simulink model "EvPowertrainController4EM"  (R2024b)
settings: configuration reference "VehicleFixed10ms" (kept outside this file)
model workspace (MAT data in the model file):
  CtrlVcuAccelPdlBpts = [0 0.8 1]
  CtrlVcuBattPnlty = 10000000
  CtrlVcuBattSOCBpts = [0 20 60 80 100]
  CtrlVcuCnstrntPnltyFctr = 10000000
  CtrlVcuEMPnlty = 100
  CtrlVcuEMTrqSplitGrid = 200
  CtrlVcuFallRate = -500
  CtrlVcuMaxAccelG = 1
  CtrlVcuMaxDecelG = -1.5
  CtrlVcuPwrDeltaPnlty = 50
  CtrlVcuPwrRatePnlty = [25 25 100]
  CtrlVcuRiseRate = 500
  CtrlVcuRoadMuEst = 0.8
  CtrlVcuSftyFctr = 0.9
  CtrlVcuTracPwrErrPnlty = 25
  CtrlVcuTrqVecBrkThresh = 0.01
  CtrlVcuTrqVecIGain = 0
  CtrlVcuTrqVecMinTrq = 25
  CtrlVcuTrqVecPGain = -2000
  CtrlVcuTrqVecSteerThresh = 0.349065850399
  CtrlVcuTrqVecVelThresh = 2.5
  N_P0 = 3
undefined symbols (not defined in the file): CtrlBcuTrlrBrkGain, CtrlVcuEvChrgLmtBpt, CtrlVcuEvRegenBrkCutOff, CtrlVcuEvRegenBrkSpdBpt, CtrlVcuEvSocBpt, eff, EnvGrvty, PlntBrkActrBoreFrnt, PlntBrkFrntBias, PlntBrkKinFricCffFrnt, PlntBrkNumPadsFrnt, PlntBrkPadMeanRadiusFrnt, PlntBrkPrsFctr, PlntBrkRearBias, PlntDiffrntl2Eff, PlntDiffrntl2Ratio, PlntDiffrntlEff, PlntDiffrntlRatio, PlntEM1EffTbl, PlntEM1Spd, PlntEM1SpdEff, PlntEM1Trq, PlntEM1TrqEff, PlntEM2EffTbl, PlntEM2Spd, PlntEM2SpdEff, PlntEM2Trq, PlntEM2TrqEff, PlntEM3EffTbl, PlntEM3Spd, PlntEM3SpdEff, PlntEM3Trq, PlntEM3TrqEff, PlntEMWhlGearEffFL, PlntEMWhlGearEffRL, PlntEMWhlGearRatioFL, PlntEMWhlGearRatioRL, PlntTransEffSpdBpt, PlntTransEffTbl, PlntTransEffTempBpt, PlntTransEffTrqBpt, PlntTransGearNumVect, PlntTransGearRatioVect, PlntVehCGHgtAxl, PlntVehDstCGFrntAxl, PlntVehDstCGRearAxl, PlntVehMass, PlntWhlLdRadiusFrnt, PlntWhlLdRadiusRear
libraries: simulink x25, autolibutils x2, slpidlib x2
(part 7 of 7)

== matlab function EvPowertrainController4EM/Torque Vectoring/Nonlinear_MPC/Nonlinear_MPCFcn ==
  data: Acc input; delta_Frnt input; TV_enableflag input; xk input; PrevEMTrqCmdFinals input; EMTrqCmds input; Vx input; EMTrqMaxFrnt input; EMTrqMaxRear input; xi_in input; EMTrqCmdFinal output; xhat_kp1 output; fval output; exitflag output; allCosts output; compTime output; stepSize output; iterations output; funcCount output; betaMax output; r_ref output; xi_out output
function [EMTrqCmdFinal, xhat_kp1, fval, exitflag, allCosts, compTime, stepSize, iterations, funcCount, betaMax, r_ref, xi_out] ...
    = Nominal_MPC(Acc, delta_Frnt, TV_enableflag, xk, PrevEMTrqCmdFinals, EMTrqCmds, Vx, EMTrqMaxFrnt, EMTrqMaxRear, xi_in)

%% MPC Tuning Parameters
Np = 10;    % prediction horizon [interval]
Nc = 3;     % control horizon [interval] 

% % -----------------------------------------------------------------

Q_y  = 150;     % Weight of yaw rate tracking
Q_du = eye(4);  % Weight of input increment (slew rate)

% % -----------------------------------------------------------------

% % % Allowed Maximum NMPC computation Iterations
Iter_max = 30;

%% Defining fixed parameter structure
nx = 2; % number of states
nu = 2; % number of controls

% % System parameters
m  = 1623;          % [kg]           % vehicle mass
Iz = 2066;          % [kg m^2]       % yaw moment of inertia
lf = 1.09;          % [m]            % distance from c.o.g. to front axle
lr = 1.7;           % [m]            % distance from c.o.g. to rear axle
lw = 1.575;         % [m]            % track width
rw = 0.309;         % [m]            % wheel radius
h  = 0.609;         % [m]            % distance from c.o.g. to ground
g  = 9.81;          % [m/s^2]        % gravitational acceleration

mu_x = 0.8*0.9;     % assumed tire-road friction coefficient

% % Tires' magic formula coefficients
D = 1.0;    % []            % peak factor scale
C = 1.1;    % []            % shape factor
E = 1.2;    % []            % curvature factor

EMWhlGearRatio = 0.98*4.1; % (wheel torque = efficiency * 4.1 * motor torque)

EMTrqIncMax = 500*0.01.*ones(4,1); % sampling time = 0.01 [s];

EMFrntTrq = EMTrqCmds(1) + EMTrqCmds(2); % front axle (motor) torque
EMRearTrq = EMTrqCmds(3) + EMTrqCmds(4); % rear  axle (motor) torque

%% System bounds
% % Bounds on input and state
u_max = [2*EMTrqMaxFrnt; 2*EMTrqMaxRear];
x_max = [Inf; Inf]; % No bounds

% % % Upper Bound on Decision Variables
xi_max = [kron(ones(Nc,1), u_max);    % control
          kron(ones(Np,1), x_max)];  % states

% % Lower Bound on Decision Variables
xi_min = [kron(ones(Nc,1), -u_max);    % control
          kron(ones(Np,1), -x_max)];  % states

% % Maximum side slip angle
Car = 2.4E4; % (estimated) rear cornering stiffness
betaMax = abs(mu_x*g*(lr/Vx^2 + m*lf/(Car*(lf+lr))));

%% Yaw rate reference
% Neutral steer
r_ref = Vx*delta_Frnt/(lf+lr);

% Maximum yaw rate reference
r_ref_max = abs(0.85* mu_x*g/Vx); 

% Saturated reference
if abs(r_ref) > r_ref_max
    r_ref = r_ref_max*sign(delta_Frnt);
end

%% Provide an initial guess by shifting the previous solution 1 step (Warm Start)
% Calculate indices for clarity
% Controls
control_end = nu*Nc;
% States
state_end   = control_end + nx*Np;

% Construct the warm start vector by shifting previous solution
xi_0 = [xi_in(nu+1 : control_end);              % shifted controls (skip first control)
        xi_in(control_end-nu+1 : control_end);  % repeat last control
        xi_in(control_end+nx+1 : state_end);    % shifted states (skip first state)
        xi_in(state_end-nx+1 : state_end)];      % repeat last state

%% Fixed parameter structure
params = struct('m',m,'Iz',Iz,'lf',lf,'lr',lr,'lw',lw,'rw',rw,'h',h,'g',g, ...
    'D', D, 'C', C, 'E', E, ...
    'Np',Np,'Nc',Nc, ...
    'Q_y',Q_y,'Q_du',Q_du, ...
    'mu_x',mu_x, 'EMTrqIncMax', EMTrqIncMax, 'EMWhlGearRatio',EMWhlGearRatio, ...
    'control_end', control_end, 'state_end', state_end);

%% MPC Call

% % Solver settings
nmpc_options = optimoptions('fmincon', 'Algorithm', 'sqp', 'MaxIterations',Iter_max, 'ScaleProblem',true);

% % % If Torque Vectoring is enable, use MPC
if TV_enableflag > 0.5

    timeStart = tic;
    [xi_out, fval, exitflag, output] = fmincon(@(xi_seq) sum(MPC_getCosts(xi_seq, xk, PrevEMTrqCmdFinals, ...
                                                EMFrntTrq, EMRearTrq, r_ref, params)),...
             xi_0, ...
             [], ...          % 
             [], ...          % 
             [], ...          % 
             [], ...          % 
             xi_min, ...
             xi_max, ...
             @(xi_seq) MPC_getConstraints(xi_seq, xk, PrevEMTrqCmdFinals, Vx, delta_Frnt, ...
                                EMTrqMaxFrnt, EMTrqMaxRear, Acc, EMFrntTrq, EMRearTrq, params), ...
             nmpc_options);

    compTime = toc(timeStart); % 0        
    % NOTE: Using tic-toc to measure computation time ONLY IF NECESSARY
    % MATLAB advises not to use tic-toc with code generation.
    % tic-toc code gen is different from the normal MATLAB code gen. 
    % They later cause problems for other control variants (PID subsystem and No Torque Vectoring subsystem)  
    
    % % Extract optimal controls
    EMTrqCmdFinal = getEMTrqs(EMFrntTrq, EMRearTrq, xi_out(1:nu));

    % % Obtain optimal (predicted) next state
    xhat_kp1 = MPC_getNextState(xk, xi_out(1:nu), EMFrntTrq, Vx, delta_Frnt, Acc, params);

    % % Acquire computed costs to examine the influence of different costs 
    allCosts = MPC_getCosts(xi_out, xk, PrevEMTrqCmdFinals, EMFrntTrq, EMRearTrq, r_ref, params);
    
    % % Last Step length by sqp
    stepSize = output.lssteplength;
    
    % % Iterations taken by fmincon
    iterations = output.iterations;

    % % Number of function evaluations
    funcCount = output.funcCount;

else    % if Torque Vectoring is not enable, use default torque commands
    EMTrqCmdFinal = EMTrqCmds;

    xi_out      = [kron(ones(Nc,1), [0;0]); % control
                   kron(ones(Np,1), xk)];      % states

    xhat_kp1    = xk;
    allCosts    = [0;0];
    exitflag    = 0;
    fval        = 0;
    compTime    = 0;
    stepSize    = 0;
    iterations  = 0;
    funcCount   = 0;
end

% % % --------------------- end of main program ----------------------


% % % ----------------------- begin of costs -----------------------

%% Cost Function
function J_vec = MPC_getCosts(xi_seq, x0, PrevEMTrqCmdFinals, EMFrntTrq, EMRearTrq, r_ref, params)
    % % Dimensions
    nx = 2;
    nu = 2;
    Nc = params.Nc;
    Np = params.Np;

    % % Initialization
    J_y         = 0;        % cost of yaw rate tracking
    J_du        = 0;        % cost of torque increment (slew rate)

    % % Extract and reshape controls from column vector (nu*Nc, 1) to matrix (nu, Nc)
    u_seq = reshape(xi_seq(1 : params.control_end), nu, Nc);

    % % Extract and reshape state sequence
    x_seq = reshape(xi_seq(params.control_end+1 : params.state_end), nx, Np);
    
    % Yaw rate tracking
    % J_y = J_y + params.Q_y*(x0(2) - r_ref)^2;
    for k = 1 : Np-1
        % Yaw rate tracking
        J_y = J_y + params.Q_y*(x_seq(2,k) - r_ref)^2;
    end
    
    % % Torque increment
    TrqInc = getEMTrqs(EMFrntTrq, EMRearTrq, u_seq(:,1)) - PrevEMTrqCmdFinals;
    J_du = J_du + TrqInc.' * params.Q_du  * TrqInc;
    %
    for k = 2 : Nc
        TrqInc = getEMTrqs(EMFrntTrq, EMRearTrq, u_seq(:,k)) ...
                    - getEMTrqs(EMFrntTrq, EMRearTrq, u_seq(:,k-1));
        J_du = J_du + TrqInc.' * params.Q_du  * TrqInc;
    end

    % % Cost vector
    J_vec = [J_y; J_du];

% end

% % % --------------------- end of costs ----------------------

% % % --------------------- begin of constraints -----------------------

%% Constraint function
function [c_ineq, c_eq] = MPC_getConstraints(xi_seq, x0, PrevEMTrqCmdFinals, ...
    Vx, delta_Frnt, EMTrqMaxFrnt, EMTrqMaxRear, Acc, EMFrntTrq, EMRearTrq, params)
    % % Dimensions
    nx = 2;
    nu = 2;
    Nc = params.Nc;
    Np = params.Np;

    % % Extract and reshape controls from column vector (nu*Nc, 1) to matrix (nu, Nc)
    u_seq = reshape(xi_seq(1 : params.control_end), nu, Nc);

    % % Extract and reshape state sequence
    x_seq = reshape(xi_seq(params.control_end+1 : params.state_end), nx, Np);
    
    % % Torque increment sequence
    EMTrqs_seq = zeros(4, Nc);
    for k = 1 : Nc
        EMTrqs_seq(:,k) = getEMTrqs(EMFrntTrq, EMRearTrq, u_seq(:,k));
    end
    EMTrqInc_seq = [EMTrqs_seq(:,1)-PrevEMTrqCmdFinals, diff(EMTrqs_seq,1,2)];

    % % -----------------------------------------------------------------
    % % % % State Continuity (SC) constraints
    c_eq_SC = nan(nx*Np,1);
    
    % State propagation
    xkp1 = MPC_getNextState(x0, u_seq(:,1), EMFrntTrq, Vx, delta_Frnt, Acc, params);
    % Continuity constraint
    c_eq_SC(1 : nx) = x_seq(:,1) - xkp1;

    for k = 2 : 1 : Nc
        % State propagation
        xkp1 = MPC_getNextState(x_seq(:,k-1), u_seq(:,k), EMFrntTrq, Vx, delta_Frnt, Acc, params);
        % Continuity constraint
        c_eq_SC(nx*(k-1)+1 : nx*(k-1)+nx) = x_seq(:,k) - xkp1;
    end

    for k = Nc+1 : 1 : Np
        % State propagation
        xkp1 = MPC_getNextState(x_seq(:,k-1), u_seq(:,Nc), EMFrntTrq, Vx, delta_Frnt, Acc, params);
        % Continuity constraint
        c_eq_SC(nx*(k-1)+1 : nx*(k-1)+nx) = x_seq(:,k) - xkp1;
    end

    % % -----------------------------------------------------------------
    % % Pure-control inequality constraint  
    c_ineq_EMTrqIncMax = nan(2*4*Nc,1); % % % Torque increment bound constraints
    c_ineq_EMTrqsMax = nan(2*4*Nc,1);  % % % Maximum allowed torque constraints
    c_ineq_vecTrq = nan(2*Nc, 1); % % % Torque vectoring encouraging constraints

    EMTrqsMax = [EMTrqMaxFrnt; EMTrqMaxFrnt; EMTrqMaxRear; EMTrqMaxRear];

    for k = 1 : Nc
        % % Maximum allowed torque increment Constraints
        c_ineq_EMTrqIncMax(2*4*(k-1)+1 : 2*4*(k-1)+2*4) = [ EMTrqInc_seq(:,k) - params.EMTrqIncMax;
                                                           -EMTrqInc_seq(:,k) - params.EMTrqIncMax ];
        % % Maximum allowed torque Constraints
        c_ineq_EMTrqsMax(2*4*(k-1)+1:2*4*(k-1)+2*4) = [ EMTrqs_seq(:,k) - EMTrqsMax;
                                                       -EMTrqs_seq(:,k) - EMTrqsMax];
        % % Vectoring torque encouragement
        c_ineq_vecTrq(2*(k-1)+1 : 2*(k-1)+2) = [-u_seq(1,k)*delta_Frnt;
                                                -u_seq(2,k)*delta_Frnt];

    end
    
    % % -----------------------------------------------------------------
    % % Inequality constraints
    c_ineq = [c_ineq_EMTrqIncMax;
              c_ineq_EMTrqsMax;
              c_ineq_vecTrq];

    % % Equality constraint
    c_eq = c_eq_SC;

% end

% % % --------------------- end of constraints ----------------------

% % % --------------------- begin of dynamics ----------------------

function xkp1 = MPC_getNextState(xk, uk, EMFrntTrq, Vx, delta_Frnt, Acc, params)
Ts = 0.01;

% % % 4th order
% k1 = MPC_getVehicleDynamics(xk, uk, EMFrntTrq, Vx, delta_Frnt, Acc, params);
% k2 = MPC_getVehicleDynamics(xk + Ts*k1/2, uk, EMFrntTrq, Vx, delta_Frnt, Acc, params);
% k3 = MPC_getVehicleDynamics(xk + Ts*k2/2, uk, EMFrntTrq, Vx, delta_Frnt, Acc,params);
% k4 = MPC_getVehicleDynamics(xk + Ts*k3, uk, EMFrntTrq, Vx, delta_Frnt, Acc, params);
% 
% xkp1 = xk + Ts*(k1 + 2*k2 + 2*k3 + k4)/6;

% % 2nd order
k1 = MPC_getVehicleDynamics(xk, uk, EMFrntTrq, Vx, delta_Frnt, Acc, params);
k2 = MPC_getVehicleDynamics(xk + Ts*k1, uk, EMFrntTrq, Vx, delta_Frnt, Acc, params);
xkp1 = xk + Ts*(k1+k2)/2;

% % 1st order
% k1 = MPC_getVehicleDynamics(xk, uk, EMFrntTrq, Vx, delta_Frnt, Acc, params);
% xkp1 = xk + Ts*k1;

% end

function xk_dot = MPC_getVehicleDynamics(xk, uk, EMFrntTrq, Vx, delta_Frnt, Acc, params)

% % System parameters
m = params.m;           % [kg]           % vehicle mass
Iz = params.Iz;         % [kg m^2]       % yaw moment of inertia
lf = params.lf;         % [m]            % distance from c.o.g. to front axle
lr = params.lr;         % [m]            % distance from c.o.g. to rear axle
lw = params.lw;         % [m]            % track width
rw = params.rw;         % [m]            % wheel radius

% Get lateral forces
[Fy, ~] = getForces(xk, Vx, delta_Frnt, Acc, params);
Fy_FL = Fy(1); Fy_FR = Fy(2); Fy_RL = Fy(3); Fy_RR = Fy(4);

% % Continuous-time dynamics
Vy_dot = ( (EMFrntTrq*params.EMWhlGearRatio/rw)*sin(delta_Frnt) + (Fy_FL+Fy_FR)*cos(delta_Frnt) + Fy_RL + Fy_RR)/m - Vx*xk(2);
r_dot  = ( ( (EMFrntTrq*params.EMWhlGearRatio/rw)*sin(delta_Frnt) + (Fy_FL+Fy_FR)*cos(delta_Frnt) )*lf ...
            + ( (uk(1)*params.EMWhlGearRatio/rw)*cos(delta_Frnt) + (Fy_FL-Fy_FR)*sin(delta_Frnt) )*lw/2 ...
            + (uk(2)*params.EMWhlGearRatio/rw)*lw/2 - (Fy_RL+Fy_RR)*lr)/Iz ;
xk_dot = [Vy_dot; r_dot];
% end

function [Fy, Fz] = getForces(xk, Vx, delta_Frnt, Acc, params)
% % System parameters
m = params.m;           % [kg]           % vehicle mass
lf = params.lf;         % [m]            % distance from c.o.g. to front axle
lr = params.lr;         % [m]            % distance from c.o.g. to rear axle
lw = params.lw;         % [m]            % track width
h  = params.h;          % [m]            % distance from c.o.g. to ground
g  = params.g;          % [m/s^2]        % gravitational acceleration
mu = params.mu_x;       % []             % friction coefficient

% % Tires' magic formula coefficients
D = params.D; % []           % peak factor scale
C = params.C; % []            % shape factor
E = params.E; % []            % curvature factor

% % Compute Vertical Loads
Fz_FL = 0.5*( m*g*lr/(lf+lr) - m*Acc(1)*h/(lf+lr) - m*-Acc(2)*h*lr/(lw*(lf+lr)) );
Fz_FR = 0.5*( m*g*lr/(lf+lr) - m*Acc(1)*h/(lf+lr) + m*-Acc(2)*h*lr/(lw*(lf+lr)) );
Fz_RL = 0.5*( m*g*lf/(lf+lr) + m*Acc(1)*h/(lf+lr) - m*-Acc(2)*h*lf/(lw*(lf+lr)) );
Fz_RR = 0.5*( m*g*lf/(lf+lr) + m*Acc(1)*h/(lf+lr) + m*-Acc(2)*h*lf/(lw*(lf+lr)) );
Fz = [Fz_FL; Fz_FR; Fz_RL; Fz_RR];

% Compute wheel side slip angles
[a_FL,a_FR,a_RL,a_RR] = getTireSlipAng(xk, Vx, delta_Frnt, params);

% % Lateral forces
Fy = [ mu*D*Fz_FL*sin( C*atan( ( 4E4/(mu*D*Fz_FL)  ) *a_FL - E*( ( 4E4/(mu*D*Fz_FL)  ) *a_FL - atan( ( 4E4/(mu*D*Fz_FL)  ) *a_FL ) ) ) );
       mu*D*Fz_FR*sin( C*atan( ( 4E4/(mu*D*Fz_FR)  ) *a_FR - E*( ( 4E4/(mu*D*Fz_FR)  ) *a_FR - atan( ( 4E4/(mu*D*Fz_FR)  ) *a_FR ) ) ) );
       mu*D*Fz_RL*sin( C*atan( ( 4E4/(mu*D*Fz_RL)  ) *a_RL - E*( ( 4E4/(mu*D*Fz_RL)  ) *a_RL - atan( ( 4E4/(mu*D*Fz_RL)  ) *a_RL ) ) ) );
       mu*D*Fz_RR*sin( C*atan( ( 4E4/(mu*D*Fz_RR)  ) *a_RR - E*( ( 4E4/(mu*D*Fz_RR)  ) *a_RR - atan( ( 4E4/(mu*D*Fz_RR)  ) *a_RR ) ) ) )    ];

% end

function [a_FL,a_FR,a_RL,a_RR] = getTireSlipAng(xk, Vx, delta_Frnt, params)
% % System parameters
lf = params.lf;         % [m]            % distance from c.o.g. to front axle
lr = params.lr;         % [m]            % distance from c.o.g. to rear axle
lw = params.lw;         % [m]            % track width

a_FL = -atan2((xk(1) + xk(2)*lf),(Vx - xk(2)*lw/2)) + delta_Frnt;        % front-left
a_FR = -atan2((xk(1) + xk(2)*lf),(Vx + xk(2)*lw/2)) + delta_Frnt;        % front-right
a_RL = -atan2((xk(1) - xk(2)*lr),(Vx - xk(2)*lw/2));                     % rear-left
a_RR = -atan2((xk(1) - xk(2)*lr),(Vx + xk(2)*lw/2));                     % rear-right

% end

function EMTrqs = getEMTrqs(EMFrntTrq, EMRearTrq, uk)
EMTrqs = [  0.5*(EMFrntTrq - uk(1)); % EMTrq_FL
            0.5*(EMFrntTrq + uk(1)); % EMTrq_FR
            0.5*(EMRearTrq - uk(2)); % EMTrq_RL
            0.5*(EMRearTrq + uk(2))  ]; % EMTrq_RR
% end

% % % --------------------- end of dynamics ----------------------

% end

== matlab function EvPowertrainController4EM/Energy Management/Hamiltonian computation and minimization/MATLAB Function ==
  data: minH output; idx output; H input; InfFlag input; allInf output
function [minH, idx, allInf] = fcn(H, InfFlag)

if all(InfFlag) 
    [minH, idx] = min(H);
    allInf = 1;
else
    [minH, idx] = min(H);
    allInf = 0;
end

== matlab function EvPowertrainController4EM/Torque Vectoring/4EM/Torque Vectoring Split Function Front ==
  data: MaxTrq input; TrqLeftOut output; TrqLeft input; TrqRght input; TrqRghtOut output; TrqVec input; Enbl input; BrkThresh input; MinTrq input
function [TrqLeftOut, TrqRghtOut] = fcn(MaxTrq, TrqLeft, TrqRght, TrqVec, Enbl, BrkThresh, MinTrq)
% Enbl:= flag to turn on TV, true if steering wheel is turned and non-zero vehicle speed
% BrkThresh:= flag to turn on TV, true if not braking
TrqLmt = min(MaxTrq-abs(TrqLeft),MaxTrq-abs(TrqRght));
DeltaTrq = min(MinTrq, min(TrqLmt,abs(TrqVec)))*sign(TrqVec)*Enbl;% limit difference in torque between tires to +/-MinTrq and to max/min motor torque
if BrkThresh > 0 % Not braking. Use Torque vectoring
    TrqLeftOut = (TrqLeft+DeltaTrq);
    TrqRghtOut = (TrqRght-DeltaTrq);
else % ignore TV
    TrqLeftOut = TrqLeft;
    TrqRghtOut = TrqRght;
end
